simulink model "encoder_reader_aksim2_complete_model"  (R2024a)
settings: Solver=FixedStepDiscrete  StartTime=0.0  StopTime=10.0  FixedStep=0.001  RelTol=1e-3
undefined symbols (not defined in the file): aksim2_error_type, encoder_error_type_t
libraries: simulink x1
settings Model: DataDictionary=enoder_dictionary.sldd  VariantFading=off  Creator=vgaggero  LastModifiedBy=jlosi
settings OptimizationCC: DefaultParameterBehavior=Inlined  EnhancedBackFolding=on  PassReuseOutputArgsAs=Individual arguments  OptimizeBlockOrder=speed  DifferentSizesBufferReuse=on  OptimizationCustomize=off  EfficientTunableParamExpr=on
settings DebuggingCC: ParameterTunabilityLossMsg=error
settings HardwareCC: ProdBitPerPointer=32  ProdBitPerSizeT=32  ProdBitPerPtrDiffT=32  ProdLargestAtomicInteger=Long  ProdLargestAtomicFloat=Double  ProdWordSize=32  ProdHWDeviceType=ARM Compatible->ARM Cortex-M
settings SFSimCC: MATLABDynamicMemAlloc=off
settings RTWCC: Description=Embedded Coder  SystemTargetFile=ert.tlc  GenCodeOnly=on  TemplateMakefile=ert_default_tmf  GPUComputeCapability=3.5
settings CodeAppCC: ForceParamTrailComments=on  IgnoreCustomStorageClasses=off  OperatorAnnotations=on  SimulinkDataObjDesc=on  SFDataObjDesc=on  InsertBlockDesc=on
settings ERTTargetCC: TargetLangStandard=C99 (ISO)  GenerateSampleERTMain=on  CodeInterfacePackaging=Reusable function  InlinedParameterPlacement=NonHierarchical  MultiInstanceErrorCode=None  RootIOFormat=Structure reference  ERTCustomFileTemplate=example_file_process.tlc

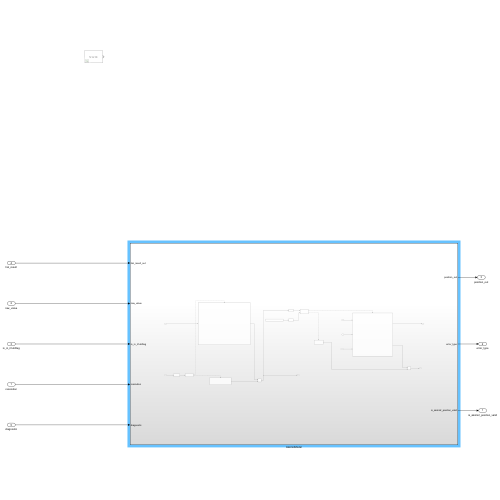
[thumbnail: Simulink's stored preview of the top-level diagram]
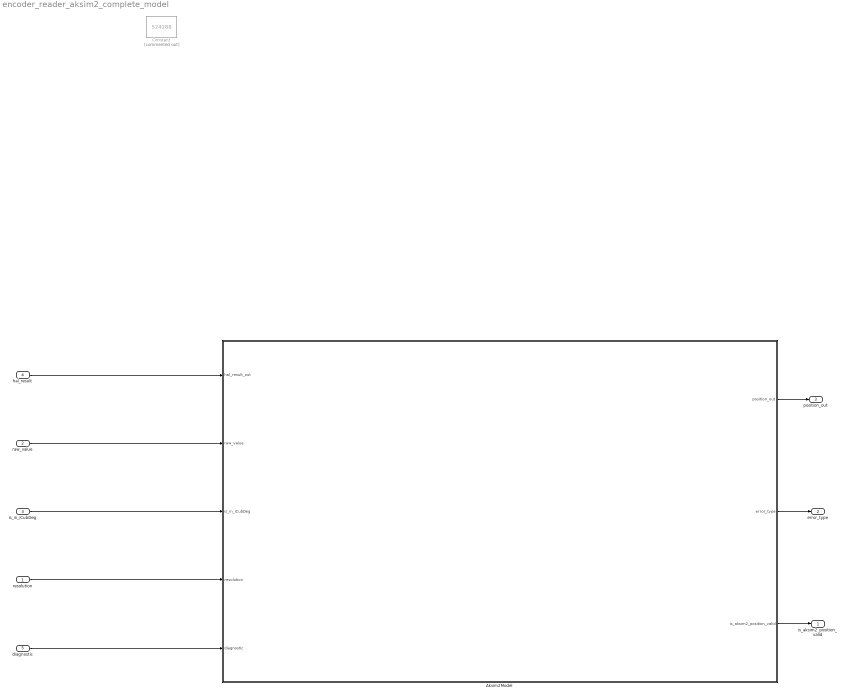
== system encoder_reader_aksim2_complete_model ==
  resolution : Inport  OutDataTypeStr=int32
  raw_value : Inport  Port=2  OutDataTypeStr=int32
  is_in_iCubDeg : Inport  Port=3  OutDataTypeStr=boolean
  hal_result : Inport  Port=4  OutDataTypeStr=Enum: hal_result_enum_t
  diagnostic : Inport  Port=5  OutDataTypeStr=Enum: aksim2_error_type
  Aksim2Model : Subsystem
  Constant : Constant  Commented=on  Value=524288
  is_aksim2_position_valid : Outport  OutDataTypeStr=boolean
  error_type : Outport  Port=2
  position_out : Outport  Port=3
  wires:
  hal_result/1 -> Aksim2Model/1(hal_result_out)
  resolution/1 -> Aksim2Model/4(resolution)
  raw_value/1 -> Aksim2Model/2(raw_value)
  is_in_iCubDeg/1 -> Aksim2Model/3(is_in_iCubDeg)
  diagnostic/1 -> Aksim2Model/5(diagnostic)
  Aksim2Model/1(position_out) -> position_out/1
  Aksim2Model/2(error_type) -> error_type/1
  Aksim2Model/3(is_aksim2_position_valid) -> is_aksim2_position_valid/1

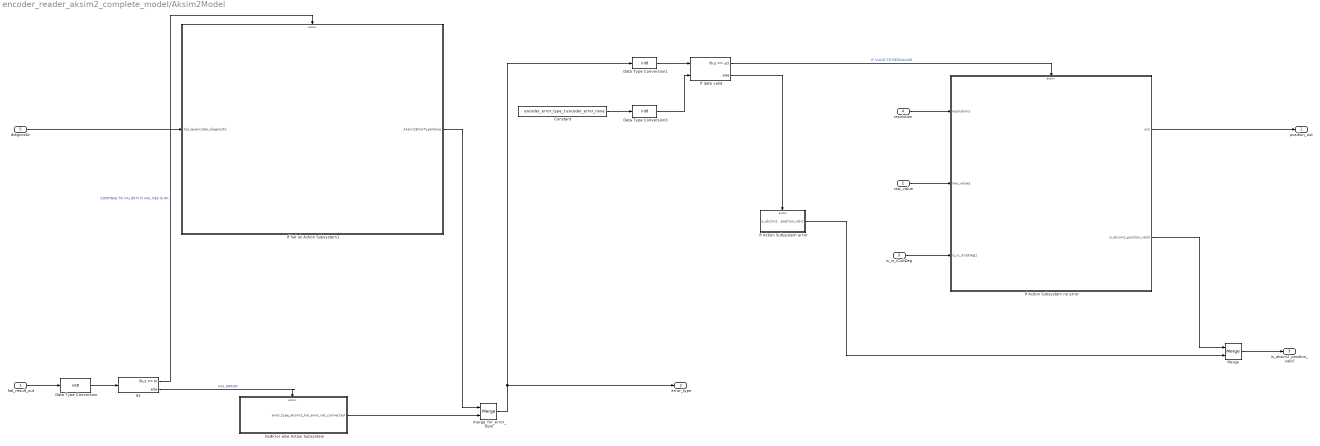
== system encoder_reader_aksim2_complete_model/Aksim2Model ==
  hal_result_out : Inport
  raw_value : Inport  Port=2
  is_in_iCubDeg : Inport  Port=3
  resolution : Inport  Port=4
  diagnostic : Inport  Port=5  OutDataTypeStr=Enum: aksim2_error_type
  Constant : Constant  Value=encoder_error_type_t.encoder_error_none  OutDataTypeStr=Enum: encoder_error_type_t
  Data Type Conversion : DataTypeConversion  OutDataTypeStr=int8  SaturateOnIntegerOverflow=off  RndMeth=Floor
  Data Type Conversion1 : DataTypeConversion  OutDataTypeStr=int8  SaturateOnIntegerOverflow=off  RndMeth=Floor
  Data Type Conversion3 : DataTypeConversion  OutDataTypeStr=int8  SaturateOnIntegerOverflow=off  RndMeth=Floor
  If Action Subsystem error : Subsystem  TreatAsAtomicUnit=on
  If Action Subsystem no error : Subsystem  TreatAsAtomicUnit=on
  If data valid : If  NumInputs=2  IfExpression=u1 == u2
  If hal ok Action Subsystem1 : Subsystem  TreatAsAtomicUnit=on
  If1 : If  IfExpression=u1 == 0
  Merge : Merge
  halError else Action Subsystem : Subsystem  TreatAsAtomicUnit=on
  merge_for_error_type : Merge
  position_out : Outport
  error_type : Outport  Port=2  OutDataTypeStr=Enum: encoder_error_type_t
  is_aksim2_position_valid : Outport  Port=3
  wires:
  resolution/1 -> If Action Subsystem no error/1(resolution1)
  If Action Subsystem no error/1(out) -> position_out/1
  raw_value/1 -> If Action Subsystem no error/2(raw_value1)
  is_in_iCubDeg/1 -> If Action Subsystem no error/3(is_in_iCubDeg1)
  hal_result_out/1 -> Data Type Conversion/1
  If1/1 -> If hal ok Action Subsystem1/Action  "CONTINUE TO VALIDITY IF HAL RES IS OK"
  If1/2 -> halError else Action Subsystem/Action  "HAL ERROR"
  Data Type Conversion/1 -> If1/1
  merge_for_error_type/1 -> error_type/1, Data Type Conversion1/1
  halError else Action Subsystem/1(error_type_aksim2_hal_error_not_connected) -> merge_for_error_type/2
  If hal ok Action Subsystem1/1(Aksim2ErrorTypeValue) -> merge_for_error_type/1
  diagnostic/1 -> If hal ok Action Subsystem1/1(hal_spiencoder_diagnostic)
  If Action Subsystem error/1(is_aksim2_position_valid) -> Merge/2
  If Action Subsystem no error/2(is_aksim2_position_valid) -> Merge/1
  Merge/1 -> is_aksim2_position_valid/1
  If data valid/2 -> If Action Subsystem error/Action
  If data valid/1 -> If Action Subsystem no error/Action  "IF VALID TO RESCAILING"
  Constant/1 -> Data Type Conversion3/1
  Data Type Conversion1/1 -> If data valid/1
  Data Type Conversion3/1 -> If data valid/2

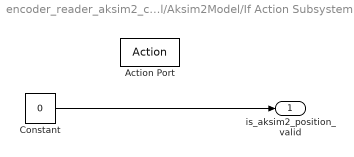
== system encoder_reader_aksim2_complete_model/Aksim2Model/If Action Subsystem error ==
  Action Port : ActionPort  ActionPortLabel=else
  Constant : Constant  Value=0  OutDataTypeStr=boolean
  is_aksim2_position_valid : Outport  OutDataTypeStr=boolean
  wires:
  Constant/1 -> is_aksim2_position_valid/1

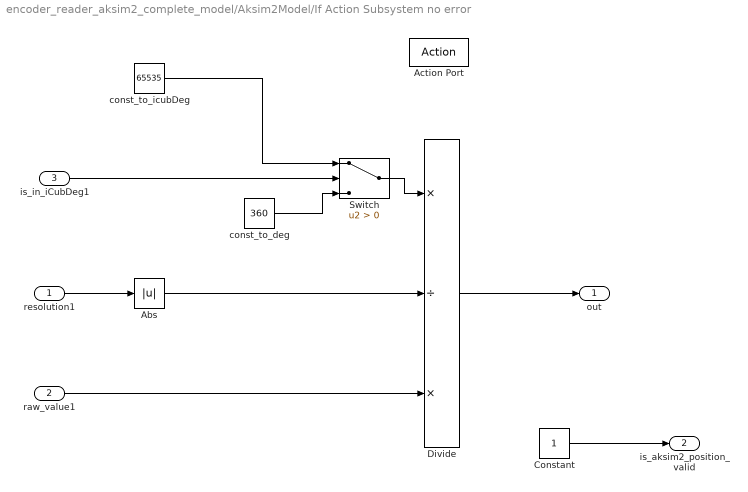
== system encoder_reader_aksim2_complete_model/Aksim2Model/If Action Subsystem no error ==
  resolution1 : Inport  OutDataTypeStr=int32
  raw_value1 : Inport  Port=2  OutDataTypeStr=int32
  is_in_iCubDeg1 : Inport  Port=3  OutDataTypeStr=boolean
  Action Port : ActionPort  ActionPortLabel=if(u1 == u2)
  Abs : Abs  SaturateOnIntegerOverflow=off
  Constant : Constant  OutDataTypeStr=boolean
  Divide : Product  Inputs=*/*
  Switch : Switch  Criteria=u2 > Threshold  SaturateOnIntegerOverflow=off  InputSameDT=off
  const_to_deg : Constant  Value=360
  const_to_icubDeg : Constant  Value=65535
  out : Outport
  is_aksim2_position_valid : Outport  Port=2
  wires:
  Abs/1 -> Divide/2
  is_in_iCubDeg1/1 -> Switch/2
  const_to_icubDeg/1 -> Switch/1
  Switch/1 -> Divide/1
  raw_value1/1 -> Divide/3
  const_to_deg/1 -> Switch/3
  Divide/1 -> out/1
  resolution1/1 -> Abs/1
  Constant/1 -> is_aksim2_position_valid/1

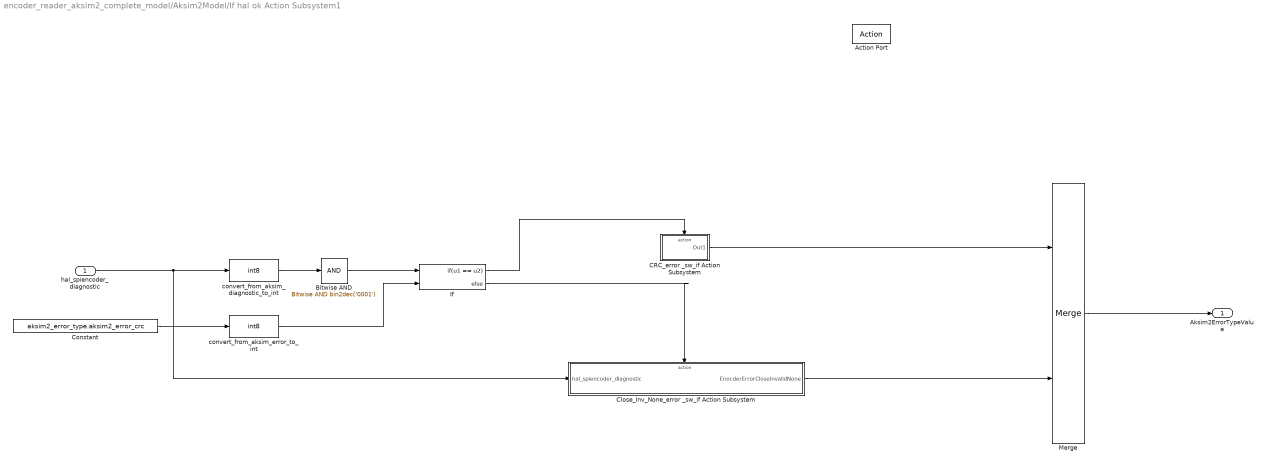
== system encoder_reader_aksim2_complete_model/Aksim2Model/If hal ok Action Subsystem1 ==
  hal_spiencoder_diagnostic : Inport
  Action Port : ActionPort  ActionPortLabel=if(u1 == 0)
  Bitwise AND : simulink/Logic and Bit Operations/Bitwise Operator  logicop=AND  UseBitMask=on  BitMask=bin2dec('0001')  BitMaskRealWorld=Stored Integer
      settings: LibrarySourceBlock=|
      | simulink/Quick Insert/Logic and Bit
      | Operations/Bitwise AND
  CRC_error _sw_if Action Subsystem : Subsystem  TreatAsAtomicUnit=on
  Close_Inv_None_error _sw_if Action Subsystem : Subsystem  TreatAsAtomicUnit=on
  Constant : Constant  Value=aksim2_error_type.aksim2_error_crc  OutDataTypeStr=Enum: aksim2_error_type
  If : If  NumInputs=2  IfExpression=u1 == u2
  Merge : Merge
  convert_from_aksim_diagnostic_to_int : DataTypeConversion  OutDataTypeStr=int8  SaturateOnIntegerOverflow=off  RndMeth=Floor
  convert_from_aksim_error_to_int : DataTypeConversion  OutDataTypeStr=int8  SaturateOnIntegerOverflow=off  RndMeth=Floor
  Aksim2ErrorTypeValue : Outport  OutDataTypeStr=Enum: encoder_error_type_t
  wires:
  Merge/1 -> Aksim2ErrorTypeValue/1
  hal_spiencoder_diagnostic/1 -> Close_Inv_None_error _sw_if Action Subsystem/1(hal_spiencoder_diagnostic), convert_from_aksim_diagnostic_to_int/1
  convert_from_aksim_diagnostic_to_int/1 -> Bitwise AND/1
  Bitwise AND/1 -> If/1
  Constant/1 -> convert_from_aksim_error_to_int/1
  convert_from_aksim_error_to_int/1 -> If/2
  If/1 -> CRC_error _sw_if Action Subsystem/Action
  CRC_error _sw_if Action Subsystem/1(Out1) -> Merge/1
  If/2 -> Close_Inv_None_error _sw_if Action Subsystem/Action
  Close_Inv_None_error _sw_if Action Subsystem/1(EnocderErrorCloseInvalidNone) -> Merge/2

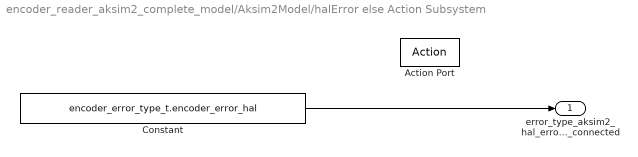
== system encoder_reader_aksim2_complete_model/Aksim2Model/halError else Action Subsystem ==
  Action Port : ActionPort  ActionPortLabel=else
  Constant : Constant  Value=encoder_error_type_t.encoder_error_hal  OutDataTypeStr=Enum: encoder_error_type_t
  error_type_aksim2_hal_error_not_connected : Outport  OutDataTypeStr=Enum: encoder_error_type_t
  wires:
  Constant/1 -> error_type_aksim2_hal_error_not_connected/1

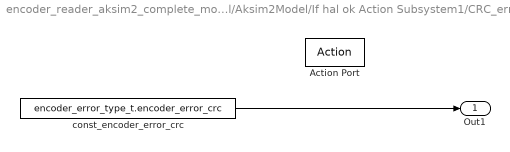
== system encoder_reader_aksim2_complete_model/Aksim2Model/If hal ok Action Subsystem1/CRC_error _sw_if Action Subsystem ==
  Action Port : ActionPort  ActionPortLabel=if(u1 == u2)
  const_encoder_error_crc : Constant  Value=encoder_error_type_t.encoder_error_crc  OutDataTypeStr=Enum: encoder_error_type_t
  Out1 : Outport
  wires:
  const_encoder_error_crc/1 -> Out1/1

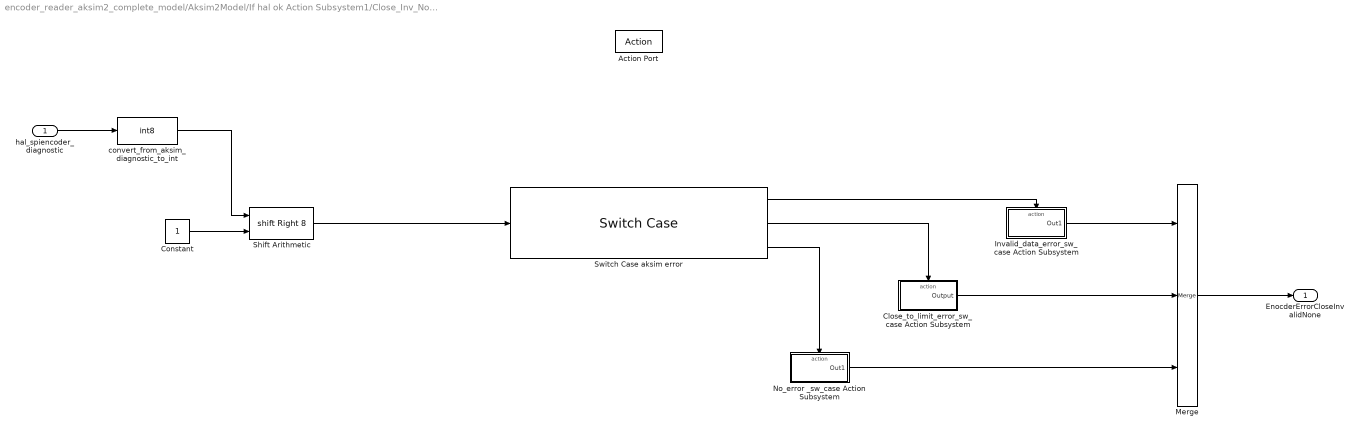
== system encoder_reader_aksim2_complete_model/Aksim2Model/If hal ok Action Subsystem1/Close_Inv_None_error _sw_if Action Subsystem ==
  hal_spiencoder_diagnostic : Inport
  Action Port : ActionPort  ActionPortLabel=else
  Close_to_limit_error_sw_case Action Subsystem : Subsystem  TreatAsAtomicUnit=on
  Constant : Constant  OutDataTypeStr=int8
  Invalid_data_error_sw_case Action Subsystem : Subsystem  TreatAsAtomicUnit=on
  Merge : Merge  Inputs=3
  No_error _sw_case Action Subsystem : Subsystem  TreatAsAtomicUnit=on
  Shift Arithmetic : ArithShift  BitShiftNumberSource=Input port  BitShiftNumber=8  BitShiftDirection=Right
      settings: InputPortMap=u0,p1
  Switch Case aksim error : SwitchCase  CaseConditions={[0,1], 2}
  convert_from_aksim_diagnostic_to_int : DataTypeConversion  OutDataTypeStr=int8  SaturateOnIntegerOverflow=off  RndMeth=Floor
  EnocderErrorCloseInvalidNone : Outport
  wires:
  hal_spiencoder_diagnostic/1 -> convert_from_aksim_diagnostic_to_int/1
  convert_from_aksim_diagnostic_to_int/1 -> Shift Arithmetic/1
  Constant/1 -> Shift Arithmetic/2
  Shift Arithmetic/1 -> Switch Case aksim error/1
  Switch Case aksim error/3 -> No_error _sw_case Action Subsystem/Action
  Switch Case aksim error/2 -> Close_to_limit_error_sw_case Action Subsystem/Action
  Switch Case aksim error/1 -> Invalid_data_error_sw_case Action Subsystem/Action
  Invalid_data_error_sw_case Action Subsystem/1(Out1) -> Merge/1
  Close_to_limit_error_sw_case Action Subsystem/1(Output) -> Merge/2
  No_error _sw_case Action Subsystem/1(Out1) -> Merge/3
  Merge/1 -> EnocderErrorCloseInvalidNone/1

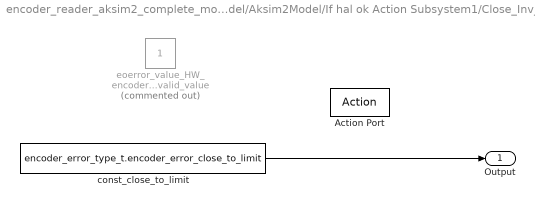
== system encoder_reader_aksim2_complete_model/Aksim2Model/If hal ok Action Subsystem1/Close_Inv_None_error _sw_if Action Subsystem/Close_to_limit_error_sw_case Action Subsystem ==
  Action Port : ActionPort  ActionPortLabel=case [ 2 ]:
  const_close_to_limit : Constant  Value=encoder_error_type_t.encoder_error_close_to_limit  OutDataTypeStr=Enum: encoder_error_type_t
  eoerror_value_HW_encoder_invalid_value : Constant  Commented=on
  Output : Outport  OutDataTypeStr=Enum: encoder_error_type_t
  wires:
  const_close_to_limit/1 -> Output/1

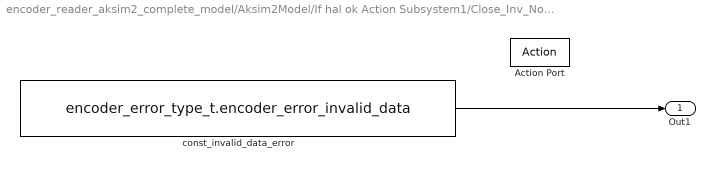
== system encoder_reader_aksim2_complete_model/Aksim2Model/If hal ok Action Subsystem1/Close_Inv_None_error _sw_if Action Subsystem/Invalid_data_error_sw_case Action Subsystem ==
  Action Port : ActionPort  ActionPortLabel=case [ 0 1 ]:
  const_invalid_data_error : Constant  Value=encoder_error_type_t.encoder_error_invalid_data  OutDataTypeStr=Enum: encoder_error_type_t
  Out1 : Outport
  wires:
  const_invalid_data_error/1 -> Out1/1

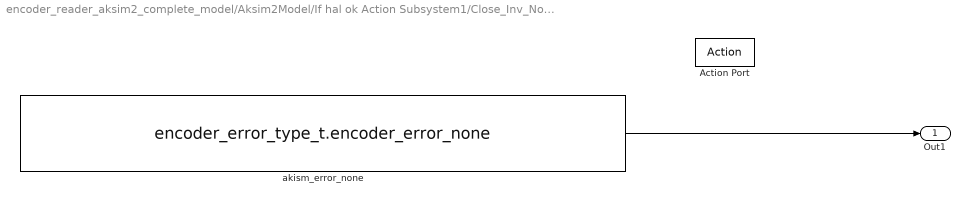
== system encoder_reader_aksim2_complete_model/Aksim2Model/If hal ok Action Subsystem1/Close_Inv_None_error _sw_if Action Subsystem/No_error _sw_case Action Subsystem ==
  Action Port : ActionPort  ActionPortLabel=default:
  akism_error_none : Constant  Value=encoder_error_type_t.encoder_error_none  OutDataTypeStr=Enum: encoder_error_type_t
  Out1 : Outport  OutDataTypeStr=Enum: encoder_error_type_t
  wires:
  akism_error_none/1 -> Out1/1
